simulink library "AtomicLibrary"
PostLoadFcn:
  | PacketBusGenerator; RailCabBusGenerator
(part 1 of 8)

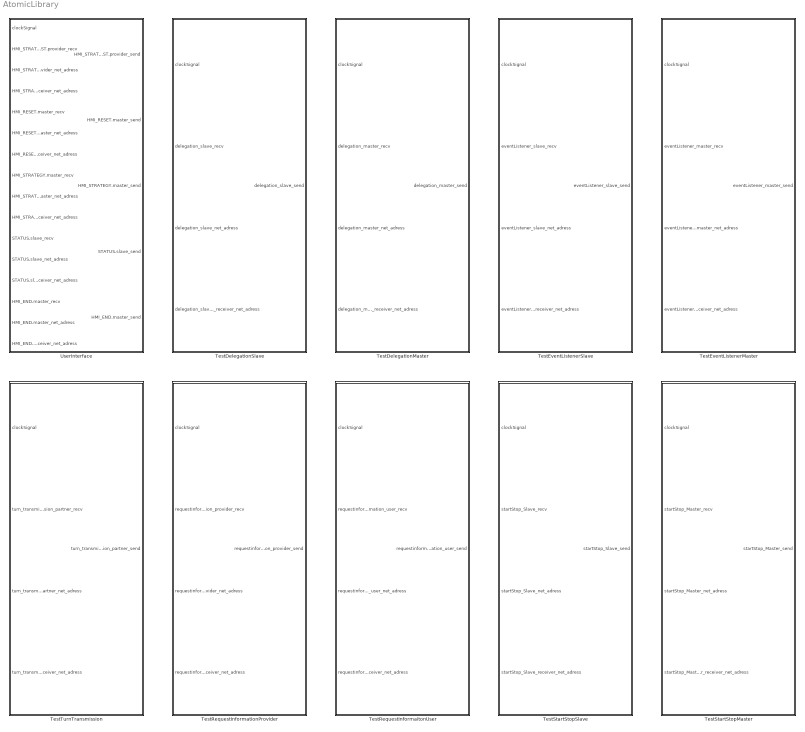
== system AtomicLibrary ==
  UserInterface : Subsystem  Tag=id=_qU3SQPdmEeGH_6eRdlYQdA
  TestDelegationSlave : Subsystem  Tag=id=_qXBOYPdmEeGH_6eRdlYQdA
  TestDelegationMaster : Subsystem  Tag=id=_qXK_YPdmEeGH_6eRdlYQdA
  TestEventListenerSlave : Subsystem  Tag=id=_qXV-gPdmEeGH_6eRdlYQdA
  TestEventListenerMaster : Subsystem  Tag=id=_qXgWkPdmEeGH_6eRdlYQdA
  TestTurnTransmission : Subsystem  Tag=id=_qXqHkPdmEeGH_6eRdlYQdA
  TestRequestInformationProvider : Subsystem  Tag=id=_qX1GsPdmEeGH_6eRdlYQdA
  TestRequestInformaitonUser : Subsystem  Tag=id=_qX_ewPdmEeGH_6eRdlYQdA
  TestStartStopSlave : Subsystem  Tag=id=_qYNhMPdmEeGH_6eRdlYQdA
  TestStartStopMaster : Subsystem  Tag=id=_qYYgUPdmEeGH_6eRdlYQdA

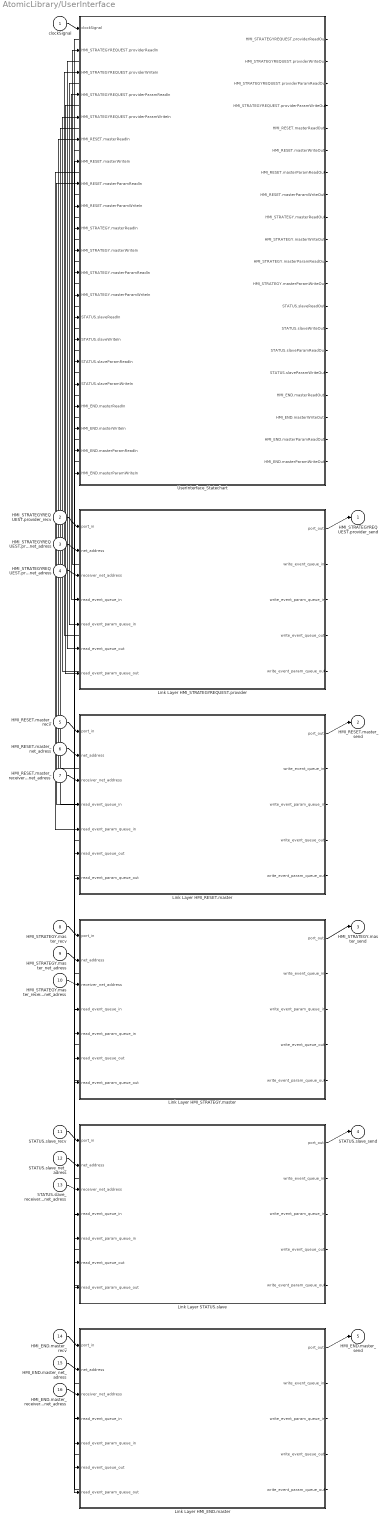
== system AtomicLibrary/UserInterface ==
  clockSignal : Inport  Tag=id=_qWKSwPdmEeGH_6eRdlYQdA  Port=1  DataType=auto  OutDataType=fixdt(1, 16)  OutScaling=2^0  OutDataTypeStr=Inherit: auto
  HMI_STRATEGYREQUEST.provider_recv : Inport  Tag=id=_r0Kh0PdmEeGH_6eRdlYQdA  Port=2  DataType=auto  OutDataType=fixdt(1, 16)  OutScaling=2^0  OutDataTypeStr=Inherit: auto
  HMI_STRATEGYREQUEST.provider_net_adress : Inport  Tag=id=_r0M-EPdmEeGH_6eRdlYQdA  Port=3  DataType=auto  OutDataType=fixdt(1, 16)  OutScaling=2^0  OutDataTypeStr=Inherit: auto
  HMI_STRATEGYREQUEST.provider_receiver_net_adress : Inport  Tag=id=_r0NlIPdmEeGH_6eRdlYQdA  Port=4  DataType=auto  OutDataType=fixdt(1, 16)  OutScaling=2^0  OutDataTypeStr=Inherit: auto
  HMI_RESET.master_recv : Inport  Tag=id=_r-XmsPdmEeGH_6eRdlYQdA  Port=5  DataType=auto  OutDataType=fixdt(1, 16)  OutScaling=2^0  OutDataTypeStr=Inherit: auto
  HMI_RESET.master_net_adress : Inport  Tag=id=_r-aC8PdmEeGH_6eRdlYQdA  Port=6  DataType=auto  OutDataType=fixdt(1, 16)  OutScaling=2^0  OutDataTypeStr=Inherit: auto
  HMI_RESET.master_receiver_net_adress : Inport  Tag=id=_r-aqAPdmEeGH_6eRdlYQdA  Port=7  DataType=auto  OutDataType=fixdt(1, 16)  OutScaling=2^0  OutDataTypeStr=Inherit: auto
  HMI_STRATEGY.master_recv : Inport  Tag=id=_sId94PdmEeGH_6eRdlYQdA  Port=8  DataType=auto  OutDataType=fixdt(1, 16)  OutScaling=2^0  OutDataTypeStr=Inherit: auto
  HMI_STRATEGY.master_net_adress : Inport  Tag=id=_sIhoQPdmEeGH_6eRdlYQdA  Port=9  DataType=auto  OutDataType=fixdt(1, 16)  OutScaling=2^0  OutDataTypeStr=Inherit: auto
  HMI_STRATEGY.master_receiver_net_adress : Inport  Tag=id=_sIi2YPdmEeGH_6eRdlYQdA  Port=10  DataType=auto  OutDataType=fixdt(1, 16)  OutScaling=2^0  OutDataTypeStr=Inherit: auto
  STATUS.slave_recv : Inport  Tag=id=_sS5sQPdmEeGH_6eRdlYQdA  Port=11  DataType=auto  OutDataType=fixdt(1, 16)  OutScaling=2^0  OutDataTypeStr=Inherit: auto
  STATUS.slave_net_adress : Inport  Tag=id=_sS8vkPdmEeGH_6eRdlYQdA  Port=12  DataType=auto  OutDataType=fixdt(1, 16)  OutScaling=2^0  OutDataTypeStr=Inherit: auto
  STATUS.slave_receiver_net_adress : Inport  Tag=id=_sS9WoPdmEeGH_6eRdlYQdA  Port=13  DataType=auto  OutDataType=fixdt(1, 16)  OutScaling=2^0  OutDataTypeStr=Inherit: auto
  HMI_END.master_recv : Inport  Tag=id=_sc4usPdmEeGH_6eRdlYQdA  Port=14  DataType=auto  OutDataType=fixdt(1, 16)  OutScaling=2^0  OutDataTypeStr=Inherit: auto
  HMI_END.master_net_adress : Inport  Tag=id=_sc7K8PdmEeGH_6eRdlYQdA  Port=15  DataType=auto  OutDataType=fixdt(1, 16)  OutScaling=2^0  OutDataTypeStr=Inherit: auto
  HMI_END.master_receiver_net_adress : Inport  Tag=id=_sc7yAPdmEeGH_6eRdlYQdA  Port=16  DataType=auto  OutDataType=fixdt(1, 16)  OutScaling=2^0  OutDataTypeStr=Inherit: auto
  HMI_STRATEGYREQUEST.provider_send : Outport  Tag=id=_r0J6wPdmEeGH_6eRdlYQdA  Port=1  DataType=auto  OutDataType=fixdt(1, 16)  OutScaling=2^0  OutDataTypeStr=Inherit: auto
  HMI_RESET.master_send : Outport  Tag=id=_r-W_oPdmEeGH_6eRdlYQdA  Port=2  DataType=auto  OutDataType=fixdt(1, 16)  OutScaling=2^0  OutDataTypeStr=Inherit: auto
  HMI_STRATEGY.master_send : Outport  Tag=id=_sIcvwPdmEeGH_6eRdlYQdA  Port=3  DataType=auto  OutDataType=fixdt(1, 16)  OutScaling=2^0  OutDataTypeStr=Inherit: auto
  STATUS.slave_send : Outport  Tag=id=_sS5FMPdmEeGH_6eRdlYQdA  Port=4  DataType=auto  OutDataType=fixdt(1, 16)  OutScaling=2^0  OutDataTypeStr=Inherit: auto
  HMI_END.master_send : Outport  Tag=id=_sc4HoPdmEeGH_6eRdlYQdA  Port=5  DataType=auto  OutDataType=fixdt(1, 16)  OutScaling=2^0  OutDataTypeStr=Inherit: auto
  Link Layer HMI_STRATEGYREQUEST.provider : Subsystem  Tag=id=_r0MXBPdmEeGH_6eRdlYQdA
  Link Layer HMI_RESET.master : Subsystem  Tag=id=_r-Zb4_dmEeGH_6eRdlYQdA
  Link Layer HMI_STRATEGY.master : Subsystem  Tag=id=_sIgaIfdmEeGH_6eRdlYQdA
  Link Layer STATUS.slave : Subsystem  Tag=id=_sS7hdPdmEeGH_6eRdlYQdA
  Link Layer HMI_END.master : Subsystem  Tag=id=_sc6j4fdmEeGH_6eRdlYQdA
  UserInterface_Statechart : Stateflow chart  Tag=id=_qVXokPdmEeGH_6eRdlYQdA
  wires:
  clockSignal/1 -> UserInterface_Statechart/1(clockSignal)
  Link Layer HMI_STRATEGYREQUEST.provider/1(port_out) -> HMI_STRATEGYREQUEST.provider_send/1
  HMI_STRATEGYREQUEST.provider_recv/1 -> Link Layer HMI_STRATEGYREQUEST.provider/1(port_in)
  UserInterface_Statechart/1(HMI_STRATEGYREQUEST.providerReadOut) -> Link Layer HMI_STRATEGYREQUEST.provider/4(read_event_queue_in)
  Link Layer HMI_STRATEGYREQUEST.provider/2(write_event_queue_in) -> UserInterface_Statechart/2(HMI_STRATEGYREQUEST.providerReadIn)
  Link Layer HMI_STRATEGYREQUEST.provider/3(write_event_param_queue_in) -> UserInterface_Statechart/4(HMI_STRATEGYREQUEST.providerParamReadIn)
  UserInterface_Statechart/3(HMI_STRATEGYREQUEST.providerParamReadOut) -> Link Layer HMI_STRATEGYREQUEST.provider/5(read_event_param_queue_in)
  UserInterface_Statechart/2(HMI_STRATEGYREQUEST.providerWriteOut) -> Link Layer HMI_STRATEGYREQUEST.provider/6(read_event_queue_out)
  UserInterface_Statechart/4(HMI_STRATEGYREQUEST.providerParamWriteOut) -> Link Layer HMI_STRATEGYREQUEST.provider/7(read_event_param_queue_out)
  Link Layer HMI_STRATEGYREQUEST.provider/4(write_event_queue_out) -> UserInterface_Statechart/3(HMI_STRATEGYREQUEST.providerWriteIn)
  Link Layer HMI_STRATEGYREQUEST.provider/5(write_event_param_queue_out) -> UserInterface_Statechart/5(HMI_STRATEGYREQUEST.providerParamWriteIn)
  HMI_STRATEGYREQUEST.provider_net_adress/1 -> Link Layer HMI_STRATEGYREQUEST.provider/2(net_address)
  HMI_STRATEGYREQUEST.provider_receiver_net_adress/1 -> Link Layer HMI_STRATEGYREQUEST.provider/3(receiver_net_address)
  Link Layer HMI_RESET.master/1(port_out) -> HMI_RESET.master_send/1
  HMI_RESET.master_recv/1 -> Link Layer HMI_RESET.master/1(port_in)
  UserInterface_Statechart/5(HMI_RESET.masterReadOut) -> Link Layer HMI_RESET.master/4(read_event_queue_in)
  Link Layer HMI_RESET.master/2(write_event_queue_in) -> UserInterface_Statechart/6(HMI_RESET.masterReadIn)
  Link Layer HMI_RESET.master/3(write_event_param_queue_in) -> UserInterface_Statechart/8(HMI_RESET.masterParamReadIn)
  UserInterface_Statechart/7(HMI_RESET.masterParamReadOut) -> Link Layer HMI_RESET.master/5(read_event_param_queue_in)
  UserInterface_Statechart/6(HMI_RESET.masterWriteOut) -> Link Layer HMI_RESET.master/6(read_event_queue_out)
  UserInterface_Statechart/8(HMI_RESET.masterParamWriteOut) -> Link Layer HMI_RESET.master/7(read_event_param_queue_out)
  Link Layer HMI_RESET.master/4(write_event_queue_out) -> UserInterface_Statechart/7(HMI_RESET.masterWriteIn)
  Link Layer HMI_RESET.master/5(write_event_param_queue_out) -> UserInterface_Statechart/9(HMI_RESET.masterParamWriteIn)
  HMI_RESET.master_net_adress/1 -> Link Layer HMI_RESET.master/2(net_address)
  HMI_RESET.master_receiver_net_adress/1 -> Link Layer HMI_RESET.master/3(receiver_net_address)
  Link Layer HMI_STRATEGY.master/1(port_out) -> HMI_STRATEGY.master_send/1
  HMI_STRATEGY.master_recv/1 -> Link Layer HMI_STRATEGY.master/1(port_in)
  UserInterface_Statechart/9(HMI_STRATEGY.masterReadOut) -> Link Layer HMI_STRATEGY.master/4(read_event_queue_in)
  Link Layer HMI_STRATEGY.master/2(write_event_queue_in) -> UserInterface_Statechart/10(HMI_STRATEGY.masterReadIn)
  Link Layer HMI_STRATEGY.master/3(write_event_param_queue_in) -> UserInterface_Statechart/12(HMI_STRATEGY.masterParamReadIn)
  UserInterface_Statechart/11(HMI_STRATEGY.masterParamReadOut) -> Link Layer HMI_STRATEGY.master/5(read_event_param_queue_in)
  UserInterface_Statechart/10(HMI_STRATEGY.masterWriteOut) -> Link Layer HMI_STRATEGY.master/6(read_event_queue_out)
  UserInterface_Statechart/12(HMI_STRATEGY.masterParamWriteOut) -> Link Layer HMI_STRATEGY.master/7(read_event_param_queue_out)
  Link Layer HMI_STRATEGY.master/4(write_event_queue_out) -> UserInterface_Statechart/11(HMI_STRATEGY.masterWriteIn)
  Link Layer HMI_STRATEGY.master/5(write_event_param_queue_out) -> UserInterface_Statechart/13(HMI_STRATEGY.masterParamWriteIn)
  HMI_STRATEGY.master_net_adress/1 -> Link Layer HMI_STRATEGY.master/2(net_address)
  HMI_STRATEGY.master_receiver_net_adress/1 -> Link Layer HMI_STRATEGY.master/3(receiver_net_address)
  Link Layer STATUS.slave/1(port_out) -> STATUS.slave_send/1
  STATUS.slave_recv/1 -> Link Layer STATUS.slave/1(port_in)
  UserInterface_Statechart/13(STATUS.slaveReadOut) -> Link Layer STATUS.slave/4(read_event_queue_in)
  Link Layer STATUS.slave/2(write_event_queue_in) -> UserInterface_Statechart/14(STATUS.slaveReadIn)
  Link Layer STATUS.slave/3(write_event_param_queue_in) -> UserInterface_Statechart/16(STATUS.slaveParamReadIn)
  UserInterface_Statechart/15(STATUS.slaveParamReadOut) -> Link Layer STATUS.slave/5(read_event_param_queue_in)
  UserInterface_Statechart/14(STATUS.slaveWriteOut) -> Link Layer STATUS.slave/6(read_event_queue_out)
  UserInterface_Statechart/16(STATUS.slaveParamWriteOut) -> Link Layer STATUS.slave/7(read_event_param_queue_out)
  Link Layer STATUS.slave/4(write_event_queue_out) -> UserInterface_Statechart/15(STATUS.slaveWriteIn)
  Link Layer STATUS.slave/5(write_event_param_queue_out) -> UserInterface_Statechart/17(STATUS.slaveParamWriteIn)
  STATUS.slave_net_adress/1 -> Link Layer STATUS.slave/2(net_address)
  STATUS.slave_receiver_net_adress/1 -> Link Layer STATUS.slave/3(receiver_net_address)
  Link Layer HMI_END.master/1(port_out) -> HMI_END.master_send/1
  HMI_END.master_recv/1 -> Link Layer HMI_END.master/1(port_in)
  UserInterface_Statechart/17(HMI_END.masterReadOut) -> Link Layer HMI_END.master/4(read_event_queue_in)
  Link Layer HMI_END.master/2(write_event_queue_in) -> UserInterface_Statechart/18(HMI_END.masterReadIn)
  Link Layer HMI_END.master/3(write_event_param_queue_in) -> UserInterface_Statechart/20(HMI_END.masterParamReadIn)
  UserInterface_Statechart/19(HMI_END.masterParamReadOut) -> Link Layer HMI_END.master/5(read_event_param_queue_in)
  UserInterface_Statechart/18(HMI_END.masterWriteOut) -> Link Layer HMI_END.master/6(read_event_queue_out)
  UserInterface_Statechart/20(HMI_END.masterParamWriteOut) -> Link Layer HMI_END.master/7(read_event_param_queue_out)
  Link Layer HMI_END.master/4(write_event_queue_out) -> UserInterface_Statechart/19(HMI_END.masterWriteIn)
  Link Layer HMI_END.master/5(write_event_param_queue_out) -> UserInterface_Statechart/21(HMI_END.masterParamWriteIn)
  HMI_END.master_net_adress/1 -> Link Layer HMI_END.master/2(net_address)
  HMI_END.master_receiver_net_adress/1 -> Link Layer HMI_END.master/3(receiver_net_address)

== system AtomicLibrary/TestDelegationSlave ==
  clockSignal : Inport  Tag=id=_qXCcgfdmEeGH_6eRdlYQdA  Port=1  DataType=auto  OutDataType=fixdt(1, 16)  OutScaling=2^0  OutDataTypeStr=Inherit: auto
  delegation_slave_recv : Inport  Tag=id=_qhxF0PdmEeGH_6eRdlYQdA  Port=2  DataType=auto  OutDataType=fixdt(1, 16)  OutScaling=2^0  OutDataTypeStr=Inherit: auto
  delegation_slave_net_adress : Inport  Tag=id=_qhziEPdmEeGH_6eRdlYQdA  Port=3  DataType=auto  OutDataType=fixdt(1, 16)  OutScaling=2^0  OutDataTypeStr=Inherit: auto
  delegation_slave_receiver_net_adress : Inport  Tag=id=_qh0JIPdmEeGH_6eRdlYQdA  Port=4  DataType=auto  OutDataType=fixdt(1, 16)  OutScaling=2^0  OutDataTypeStr=Inherit: auto
  delegation_slave_send : Outport  Tag=id=_qhwewPdmEeGH_6eRdlYQdA  Port=1  DataType=auto  OutDataType=fixdt(1, 16)  OutScaling=2^0  OutDataTypeStr=Inherit: auto
  Link Layer delegation_slave : Subsystem  Tag=id=_qhy7A_dmEeGH_6eRdlYQdA
  TestDelegationSlave_Statechart : Stateflow chart  Tag=id=_qXB1cPdmEeGH_6eRdlYQdA
  wires:
  clockSignal/1 -> TestDelegationSlave_Statechart/1(clockSignal)
  Link Layer delegation_slave/1(port_out) -> delegation_slave_send/1
  delegation_slave_recv/1 -> Link Layer delegation_slave/1(port_in)
  TestDelegationSlave_Statechart/1(delegation_slaveReadOut) -> Link Layer delegation_slave/4(read_event_queue_in)
  Link Layer delegation_slave/2(write_event_queue_in) -> TestDelegationSlave_Statechart/2(delegation_slaveReadIn)
  Link Layer delegation_slave/3(write_event_param_queue_in) -> TestDelegationSlave_Statechart/4(delegation_slaveParamReadIn)
  TestDelegationSlave_Statechart/3(delegation_slaveParamReadOut) -> Link Layer delegation_slave/5(read_event_param_queue_in)
  TestDelegationSlave_Statechart/2(delegation_slaveWriteOut) -> Link Layer delegation_slave/6(read_event_queue_out)
  TestDelegationSlave_Statechart/4(delegation_slaveParamWriteOut) -> Link Layer delegation_slave/7(read_event_param_queue_out)
  Link Layer delegation_slave/4(write_event_queue_out) -> TestDelegationSlave_Statechart/3(delegation_slaveWriteIn)
  Link Layer delegation_slave/5(write_event_param_queue_out) -> TestDelegationSlave_Statechart/5(delegation_slaveParamWriteIn)
  delegation_slave_net_adress/1 -> Link Layer delegation_slave/2(net_address)
  delegation_slave_receiver_net_adress/1 -> Link Layer delegation_slave/3(receiver_net_address)

== system AtomicLibrary/TestDelegationMaster ==
  clockSignal : Inport  Tag=id=_qXMNgfdmEeGH_6eRdlYQdA  Port=1  DataType=auto  OutDataType=fixdt(1, 16)  OutScaling=2^0  OutDataTypeStr=Inherit: auto
  delegation_master_recv : Inport  Tag=id=_qrRnIPdmEeGH_6eRdlYQdA  Port=2  DataType=auto  OutDataType=fixdt(1, 16)  OutScaling=2^0  OutDataTypeStr=Inherit: auto
  delegation_master_net_adress : Inport  Tag=id=_qrUDYPdmEeGH_6eRdlYQdA  Port=3  DataType=auto  OutDataType=fixdt(1, 16)  OutScaling=2^0  OutDataTypeStr=Inherit: auto
  delegation_master_receiver_net_adress : Inport  Tag=id=_qrUqcPdmEeGH_6eRdlYQdA  Port=4  DataType=auto  OutDataType=fixdt(1, 16)  OutScaling=2^0  OutDataTypeStr=Inherit: auto
  delegation_master_send : Outport  Tag=id=_qrRAEPdmEeGH_6eRdlYQdA  Port=1  DataType=auto  OutDataType=fixdt(1, 16)  OutScaling=2^0  OutDataTypeStr=Inherit: auto
  Link Layer delegation_master : Subsystem  Tag=id=_qrTcU_dmEeGH_6eRdlYQdA
  TestDelegationMaster_Statechart : Stateflow chart  Tag=id=_qXLmcPdmEeGH_6eRdlYQdA
  wires:
  clockSignal/1 -> TestDelegationMaster_Statechart/1(clockSignal)
  Link Layer delegation_master/1(port_out) -> delegation_master_send/1
  delegation_master_recv/1 -> Link Layer delegation_master/1(port_in)
  TestDelegationMaster_Statechart/1(delegation_masterReadOut) -> Link Layer delegation_master/4(read_event_queue_in)
  Link Layer delegation_master/2(write_event_queue_in) -> TestDelegationMaster_Statechart/2(delegation_masterReadIn)
  Link Layer delegation_master/3(write_event_param_queue_in) -> TestDelegationMaster_Statechart/4(delegation_masterParamReadIn)
  TestDelegationMaster_Statechart/3(delegation_masterParamReadOut) -> Link Layer delegation_master/5(read_event_param_queue_in)
  TestDelegationMaster_Statechart/2(delegation_masterWriteOut) -> Link Layer delegation_master/6(read_event_queue_out)
  TestDelegationMaster_Statechart/4(delegation_masterParamWriteOut) -> Link Layer delegation_master/7(read_event_param_queue_out)
  Link Layer delegation_master/4(write_event_queue_out) -> TestDelegationMaster_Statechart/3(delegation_masterWriteIn)
  Link Layer delegation_master/5(write_event_param_queue_out) -> TestDelegationMaster_Statechart/5(delegation_masterParamWriteIn)
  delegation_master_net_adress/1 -> Link Layer delegation_master/2(net_address)
  delegation_master_receiver_net_adress/1 -> Link Layer delegation_master/3(receiver_net_address)

== system AtomicLibrary/TestEventListenerSlave ==
  clockSignal : Inport  Tag=id=_qXXMofdmEeGH_6eRdlYQdA  Port=1  DataType=auto  OutDataType=fixdt(1, 16)  OutScaling=2^0  OutDataTypeStr=Inherit: auto
  eventListener_slave_recv : Inport  Tag=id=_q0bjIPdmEeGH_6eRdlYQdA  Port=2  DataType=auto  OutDataType=fixdt(1, 16)  OutScaling=2^0  OutDataTypeStr=Inherit: auto
  eventListener_slave_net_adress : Inport  Tag=id=_q0d_YPdmEeGH_6eRdlYQdA  Port=3  DataType=auto  OutDataType=fixdt(1, 16)  OutScaling=2^0  OutDataTypeStr=Inherit: auto
  eventListener_slave_receiver_net_adress : Inport  Tag=id=_q0d_YfdmEeGH_6eRdlYQdA  Port=4  DataType=auto  OutDataType=fixdt(1, 16)  OutScaling=2^0  OutDataTypeStr=Inherit: auto
  eventListener_slave_send : Outport  Tag=id=_q0a8EPdmEeGH_6eRdlYQdA  Port=1  DataType=auto  OutDataType=fixdt(1, 16)  OutScaling=2^0  OutDataTypeStr=Inherit: auto
  Link Layer eventListener_slave : Subsystem  Tag=id=_q0dYUPdmEeGH_6eRdlYQdA
  TestEventListenerSlave_Statechart : Stateflow chart  Tag=id=_qXWlkPdmEeGH_6eRdlYQdA
  wires:
  clockSignal/1 -> TestEventListenerSlave_Statechart/1(clockSignal)
  Link Layer eventListener_slave/1(port_out) -> eventListener_slave_send/1
  eventListener_slave_recv/1 -> Link Layer eventListener_slave/1(port_in)
  TestEventListenerSlave_Statechart/1(eventListener_slaveReadOut) -> Link Layer eventListener_slave/4(read_event_queue_in)
  Link Layer eventListener_slave/2(write_event_queue_in) -> TestEventListenerSlave_Statechart/2(eventListener_slaveReadIn)
  Link Layer eventListener_slave/3(write_event_param_queue_in) -> TestEventListenerSlave_Statechart/4(eventListener_slaveParamReadIn)
  TestEventListenerSlave_Statechart/3(eventListener_slaveParamReadOut) -> Link Layer eventListener_slave/5(read_event_param_queue_in)
  TestEventListenerSlave_Statechart/2(eventListener_slaveWriteOut) -> Link Layer eventListener_slave/6(read_event_queue_out)
  TestEventListenerSlave_Statechart/4(eventListener_slaveParamWriteOut) -> Link Layer eventListener_slave/7(read_event_param_queue_out)
  Link Layer eventListener_slave/4(write_event_queue_out) -> TestEventListenerSlave_Statechart/3(eventListener_slaveWriteIn)
  Link Layer eventListener_slave/5(write_event_param_queue_out) -> TestEventListenerSlave_Statechart/5(eventListener_slaveParamWriteIn)
  eventListener_slave_net_adress/1 -> Link Layer eventListener_slave/2(net_address)
  eventListener_slave_receiver_net_adress/1 -> Link Layer eventListener_slave/3(receiver_net_address)

== system AtomicLibrary/TestEventListenerMaster ==
  clockSignal : Inport  Tag=id=_qXg9ovdmEeGH_6eRdlYQdA  Port=1  DataType=auto  OutDataType=fixdt(1, 16)  OutScaling=2^0  OutDataTypeStr=Inherit: auto
  eventListener_master_recv : Inport  Tag=id=_q9nUUPdmEeGH_6eRdlYQdA  Port=2  DataType=auto  OutDataType=fixdt(1, 16)  OutScaling=2^0  OutDataTypeStr=Inherit: auto
  eventListener_master_net_adress : Inport  Tag=id=_q9pJgPdmEeGH_6eRdlYQdA  Port=3  DataType=auto  OutDataType=fixdt(1, 16)  OutScaling=2^0  OutDataTypeStr=Inherit: auto
  eventListener_master_receiver_net_adress : Inport  Tag=id=_q9pwkPdmEeGH_6eRdlYQdA  Port=4  DataType=auto  OutDataType=fixdt(1, 16)  OutScaling=2^0  OutDataTypeStr=Inherit: auto
  eventListener_master_send : Outport  Tag=id=_q9mtQPdmEeGH_6eRdlYQdA  Port=1  DataType=auto  OutDataType=fixdt(1, 16)  OutScaling=2^0  OutDataTypeStr=Inherit: auto
  Link Layer eventListener_master : Subsystem  Tag=id=_q9oidfdmEeGH_6eRdlYQdA
  TestEventListenerMaster_Statechart : Stateflow chart  Tag=id=_qXg9oPdmEeGH_6eRdlYQdA
  wires:
  clockSignal/1 -> TestEventListenerMaster_Statechart/1(clockSignal)
  Link Layer eventListener_master/1(port_out) -> eventListener_master_send/1
  eventListener_master_recv/1 -> Link Layer eventListener_master/1(port_in)
  TestEventListenerMaster_Statechart/1(eventListener_masterReadOut) -> Link Layer eventListener_master/4(read_event_queue_in)
  Link Layer eventListener_master/2(write_event_queue_in) -> TestEventListenerMaster_Statechart/2(eventListener_masterReadIn)
  Link Layer eventListener_master/3(write_event_param_queue_in) -> TestEventListenerMaster_Statechart/4(eventListener_masterParamReadIn)
  TestEventListenerMaster_Statechart/3(eventListener_masterParamReadOut) -> Link Layer eventListener_master/5(read_event_param_queue_in)
  TestEventListenerMaster_Statechart/2(eventListener_masterWriteOut) -> Link Layer eventListener_master/6(read_event_queue_out)
  TestEventListenerMaster_Statechart/4(eventListener_masterParamWriteOut) -> Link Layer eventListener_master/7(read_event_param_queue_out)
  Link Layer eventListener_master/4(write_event_queue_out) -> TestEventListenerMaster_Statechart/3(eventListener_masterWriteIn)
  Link Layer eventListener_master/5(write_event_param_queue_out) -> TestEventListenerMaster_Statechart/5(eventListener_masterParamWriteIn)
  eventListener_master_net_adress/1 -> Link Layer eventListener_master/2(net_address)
  eventListener_master_receiver_net_adress/1 -> Link Layer eventListener_master/3(receiver_net_address)

== system AtomicLibrary/TestTurnTransmission ==
  clockSignal : Inport  Tag=id=_qXrVsfdmEeGH_6eRdlYQdA  Port=1  DataType=auto  OutDataType=fixdt(1, 16)  OutScaling=2^0  OutDataTypeStr=Inherit: auto
  turn_transmission_partner_recv : Inport  Tag=id=_rGbSEPdmEeGH_6eRdlYQdA  Port=2  DataType=auto  OutDataType=fixdt(1, 16)  OutScaling=2^0  OutDataTypeStr=Inherit: auto
  turn_transmission_partner_net_adress : Inport  Tag=id=_rGduUPdmEeGH_6eRdlYQdA  Port=3  DataType=auto  OutDataType=fixdt(1, 16)  OutScaling=2^0  OutDataTypeStr=Inherit: auto
  turn_transmission_partner_receiver_net_adress : Inport  Tag=id=_rGeVYPdmEeGH_6eRdlYQdA  Port=4  DataType=auto  OutDataType=fixdt(1, 16)  OutScaling=2^0  OutDataTypeStr=Inherit: auto
  turn_transmission_partner_send : Outport  Tag=id=_rGarAPdmEeGH_6eRdlYQdA  Port=1  DataType=auto  OutDataType=fixdt(1, 16)  OutScaling=2^0  OutDataTypeStr=Inherit: auto
  Link Layer turn_transmission_partner : Subsystem  Tag=id=_rGdHQvdmEeGH_6eRdlYQdA
  TestTurnTransmission_Statechart : Stateflow chart  Tag=id=_qXquoPdmEeGH_6eRdlYQdA
  wires:
  clockSignal/1 -> TestTurnTransmission_Statechart/1(clockSignal)
  Link Layer turn_transmission_partner/1(port_out) -> turn_transmission_partner_send/1
  turn_transmission_partner_recv/1 -> Link Layer turn_transmission_partner/1(port_in)
  TestTurnTransmission_Statechart/1(turn_transmission_partnerReadOut) -> Link Layer turn_transmission_partner/4(read_event_queue_in)
  Link Layer turn_transmission_partner/2(write_event_queue_in) -> TestTurnTransmission_Statechart/2(turn_transmission_partnerReadIn)
  Link Layer turn_transmission_partner/3(write_event_param_queue_in) -> TestTurnTransmission_Statechart/4(turn_transmission_partnerParamReadIn)
  TestTurnTransmission_Statechart/3(turn_transmission_partnerParamReadOut) -> Link Layer turn_transmission_partner/5(read_event_param_queue_in)
  TestTurnTransmission_Statechart/2(turn_transmission_partnerWriteOut) -> Link Layer turn_transmission_partner/6(read_event_queue_out)
  TestTurnTransmission_Statechart/4(turn_transmission_partnerParamWriteOut) -> Link Layer turn_transmission_partner/7(read_event_param_queue_out)
  Link Layer turn_transmission_partner/4(write_event_queue_out) -> TestTurnTransmission_Statechart/3(turn_transmission_partnerWriteIn)
  Link Layer turn_transmission_partner/5(write_event_param_queue_out) -> TestTurnTransmission_Statechart/5(turn_transmission_partnerParamWriteIn)
  turn_transmission_partner_net_adress/1 -> Link Layer turn_transmission_partner/2(net_address)
  turn_transmission_partner_receiver_net_adress/1 -> Link Layer turn_transmission_partner/3(receiver_net_address)

== system AtomicLibrary/TestRequestInformationProvider ==
  clockSignal : Inport  Tag=id=_qX2U0fdmEeGH_6eRdlYQdA  Port=1  DataType=auto  OutDataType=fixdt(1, 16)  OutScaling=2^0  OutDataTypeStr=Inherit: auto
  requestinformation_provider_recv : Inport  Tag=id=_rPfHcPdmEeGH_6eRdlYQdA  Port=2  DataType=auto  OutDataType=fixdt(1, 16)  OutScaling=2^0  OutDataTypeStr=Inherit: auto
  requestinformation_provider_net_adress : Inport  Tag=id=_rPiKwPdmEeGH_6eRdlYQdA  Port=3  DataType=auto  OutDataType=fixdt(1, 16)  OutScaling=2^0  OutDataTypeStr=Inherit: auto
  requestinformation_provider_receiver_net_adress : Inport  Tag=id=_rPjY4PdmEeGH_6eRdlYQdA  Port=4  DataType=auto  OutDataType=fixdt(1, 16)  OutScaling=2^0  OutDataTypeStr=Inherit: auto
  requestinformation_provider_send : Outport  Tag=id=_rPegYPdmEeGH_6eRdlYQdA  Port=1  DataType=auto  OutDataType=fixdt(1, 16)  OutScaling=2^0  OutDataTypeStr=Inherit: auto
  Link Layer requestinformation_provider : Subsystem  Tag=id=_rPhjsPdmEeGH_6eRdlYQdA
  TestRequestInformationProvider_Statechart : Stateflow chart  Tag=id=_qX1twPdmEeGH_6eRdlYQdA
  wires:
  clockSignal/1 -> TestRequestInformationProvider_Statechart/1(clockSignal)
  Link Layer requestinformation_provider/1(port_out) -> requestinformation_provider_send/1
  requestinformation_provider_recv/1 -> Link Layer requestinformation_provider/1(port_in)
  TestRequestInformationProvider_Statechart/1(requestinformation_providerReadOut) -> Link Layer requestinformation_provider/4(read_event_queue_in)
  Link Layer requestinformation_provider/2(write_event_queue_in) -> TestRequestInformationProvider_Statechart/2(requestinformation_providerReadIn)
  Link Layer requestinformation_provider/3(write_event_param_queue_in) -> TestRequestInformationProvider_Statechart/4(requestinformation_providerParamReadIn)
  TestRequestInformationProvider_Statechart/3(requestinformation_providerParamReadOut) -> Link Layer requestinformation_provider/5(read_event_param_queue_in)
  TestRequestInformationProvider_Statechart/2(requestinformation_providerWriteOut) -> Link Layer requestinformation_provider/6(read_event_queue_out)
  TestRequestInformationProvider_Statechart/4(requestinformation_providerParamWriteOut) -> Link Layer requestinformation_provider/7(read_event_param_queue_out)
  Link Layer requestinformation_provider/4(write_event_queue_out) -> TestRequestInformationProvider_Statechart/3(requestinformation_providerWriteIn)
  Link Layer requestinformation_provider/5(write_event_param_queue_out) -> TestRequestInformationProvider_Statechart/5(requestinformation_providerParamWriteIn)
  requestinformation_provider_net_adress/1 -> Link Layer requestinformation_provider/2(net_address)
  requestinformation_provider_receiver_net_adress/1 -> Link Layer requestinformation_provider/3(receiver_net_address)

== system AtomicLibrary/TestRequestInformaitonUser ==
  clockSignal : Inport  Tag=id=_qYAs4PdmEeGH_6eRdlYQdA  Port=1  DataType=auto  OutDataType=fixdt(1, 16)  OutScaling=2^0  OutDataTypeStr=Inherit: auto
  requestinformation_user_recv : Inport  Tag=id=_rYAxUPdmEeGH_6eRdlYQdA  Port=2  DataType=auto  OutDataType=fixdt(1, 16)  OutScaling=2^0  OutDataTypeStr=Inherit: auto
  requestinformation_user_net_adress : Inport  Tag=id=_rYCmgPdmEeGH_6eRdlYQdA  Port=3  DataType=auto  OutDataType=fixdt(1, 16)  OutScaling=2^0  OutDataTypeStr=Inherit: auto
  requestinformation_user_receiver_net_adress : Inport  Tag=id=_rYDNkPdmEeGH_6eRdlYQdA  Port=4  DataType=auto  OutDataType=fixdt(1, 16)  OutScaling=2^0  OutDataTypeStr=Inherit: auto
  requestinformation_user_send : Outport  Tag=id=_rYAKQPdmEeGH_6eRdlYQdA  Port=1  DataType=auto  OutDataType=fixdt(1, 16)  OutScaling=2^0  OutDataTypeStr=Inherit: auto
  Link Layer requestinformation_user : Subsystem  Tag=id=_rYB_dPdmEeGH_6eRdlYQdA
  TestRequestInformaitonUser_Statechart : Stateflow chart  Tag=id=_qYAF0PdmEeGH_6eRdlYQdA
  wires:
  clockSignal/1 -> TestRequestInformaitonUser_Statechart/1(clockSignal)
  Link Layer requestinformation_user/1(port_out) -> requestinformation_user_send/1
  requestinformation_user_recv/1 -> Link Layer requestinformation_user/1(port_in)
  TestRequestInformaitonUser_Statechart/1(requestinformation_userReadOut) -> Link Layer requestinformation_user/4(read_event_queue_in)
  Link Layer requestinformation_user/2(write_event_queue_in) -> TestRequestInformaitonUser_Statechart/2(requestinformation_userReadIn)
  Link Layer requestinformation_user/3(write_event_param_queue_in) -> TestRequestInformaitonUser_Statechart/4(requestinformation_userParamReadIn)
  TestRequestInformaitonUser_Statechart/3(requestinformation_userParamReadOut) -> Link Layer requestinformation_user/5(read_event_param_queue_in)
  TestRequestInformaitonUser_Statechart/2(requestinformation_userWriteOut) -> Link Layer requestinformation_user/6(read_event_queue_out)
  TestRequestInformaitonUser_Statechart/4(requestinformation_userParamWriteOut) -> Link Layer requestinformation_user/7(read_event_param_queue_out)
  Link Layer requestinformation_user/4(write_event_queue_out) -> TestRequestInformaitonUser_Statechart/3(requestinformation_userWriteIn)
  Link Layer requestinformation_user/5(write_event_param_queue_out) -> TestRequestInformaitonUser_Statechart/5(requestinformation_userParamWriteIn)
  requestinformation_user_net_adress/1 -> Link Layer requestinformation_user/2(net_address)
  requestinformation_user_receiver_net_adress/1 -> Link Layer requestinformation_user/3(receiver_net_address)

== system AtomicLibrary/TestStartStopSlave ==
  clockSignal : Inport  Tag=id=_qYOvUfdmEeGH_6eRdlYQdA  Port=1  DataType=auto  OutDataType=fixdt(1, 16)  OutScaling=2^0  OutDataTypeStr=Inherit: auto
  startStop_Slave_recv : Inport  Tag=id=_rgzg8PdmEeGH_6eRdlYQdA  Port=2  DataType=auto  OutDataType=fixdt(1, 16)  OutScaling=2^0  OutDataTypeStr=Inherit: auto
  startStop_Slave_net_adress : Inport  Tag=id=_rg19MPdmEeGH_6eRdlYQdA  Port=3  DataType=auto  OutDataType=fixdt(1, 16)  OutScaling=2^0  OutDataTypeStr=Inherit: auto
  startStop_Slave_receiver_net_adress : Inport  Tag=id=_rg2kQPdmEeGH_6eRdlYQdA  Port=4  DataType=auto  OutDataType=fixdt(1, 16)  OutScaling=2^0  OutDataTypeStr=Inherit: auto
  startStop_Slave_send : Outport  Tag=id=_rgy54PdmEeGH_6eRdlYQdA  Port=1  DataType=auto  OutDataType=fixdt(1, 16)  OutScaling=2^0  OutDataTypeStr=Inherit: auto
  Link Layer startStop_Slave : Subsystem  Tag=id=_rg1WIvdmEeGH_6eRdlYQdA
  TestStartStopSlave_Statechart : Stateflow chart  Tag=id=_qYOIQPdmEeGH_6eRdlYQdA
  wires:
  clockSignal/1 -> TestStartStopSlave_Statechart/1(clockSignal)
  Link Layer startStop_Slave/1(port_out) -> startStop_Slave_send/1
  startStop_Slave_recv/1 -> Link Layer startStop_Slave/1(port_in)
  TestStartStopSlave_Statechart/1(startStop_SlaveReadOut) -> Link Layer startStop_Slave/4(read_event_queue_in)
  Link Layer startStop_Slave/2(write_event_queue_in) -> TestStartStopSlave_Statechart/2(startStop_SlaveReadIn)
  Link Layer startStop_Slave/3(write_event_param_queue_in) -> TestStartStopSlave_Statechart/4(startStop_SlaveParamReadIn)
  TestStartStopSlave_Statechart/3(startStop_SlaveParamReadOut) -> Link Layer startStop_Slave/5(read_event_param_queue_in)
  TestStartStopSlave_Statechart/2(startStop_SlaveWriteOut) -> Link Layer startStop_Slave/6(read_event_queue_out)
  TestStartStopSlave_Statechart/4(startStop_SlaveParamWriteOut) -> Link Layer startStop_Slave/7(read_event_param_queue_out)
  Link Layer startStop_Slave/4(write_event_queue_out) -> TestStartStopSlave_Statechart/3(startStop_SlaveWriteIn)
  Link Layer startStop_Slave/5(write_event_param_queue_out) -> TestStartStopSlave_Statechart/5(startStop_SlaveParamWriteIn)
  startStop_Slave_net_adress/1 -> Link Layer startStop_Slave/2(net_address)
  startStop_Slave_receiver_net_adress/1 -> Link Layer startStop_Slave/3(receiver_net_address)

== system AtomicLibrary/TestStartStopMaster ==
  clockSignal : Inport  Tag=id=_qYaVgPdmEeGH_6eRdlYQdA  Port=1  DataType=auto  OutDataType=fixdt(1, 16)  OutScaling=2^0  OutDataTypeStr=Inherit: auto
  startStop_Master_recv : Inport  Tag=id=_rqOisPdmEeGH_6eRdlYQdA  Port=2  DataType=auto  OutDataType=fixdt(1, 16)  OutScaling=2^0  OutDataTypeStr=Inherit: auto
  startStop_Master_net_adress : Inport  Tag=id=_rqQ-8PdmEeGH_6eRdlYQdA  Port=3  DataType=auto  OutDataType=fixdt(1, 16)  OutScaling=2^0  OutDataTypeStr=Inherit: auto
  startStop_Master_receiver_net_adress : Inport  Tag=id=_rqRmAPdmEeGH_6eRdlYQdA  Port=4  DataType=auto  OutDataType=fixdt(1, 16)  OutScaling=2^0  OutDataTypeStr=Inherit: auto
  startStop_Master_send : Outport  Tag=id=_rqN7oPdmEeGH_6eRdlYQdA  Port=1  DataType=auto  OutDataType=fixdt(1, 16)  OutScaling=2^0  OutDataTypeStr=Inherit: auto
  Link Layer startStop_Master : Subsystem  Tag=id=_rqQX4_dmEeGH_6eRdlYQdA
  TestStartStopMaster_Statechart : Stateflow chart  Tag=id=_qYZucPdmEeGH_6eRdlYQdA
  wires:
  clockSignal/1 -> TestStartStopMaster_Statechart/1(clockSignal)
  Link Layer startStop_Master/1(port_out) -> startStop_Master_send/1
  startStop_Master_recv/1 -> Link Layer startStop_Master/1(port_in)
  TestStartStopMaster_Statechart/1(startStop_MasterReadOut) -> Link Layer startStop_Master/4(read_event_queue_in)
  Link Layer startStop_Master/2(write_event_queue_in) -> TestStartStopMaster_Statechart/2(startStop_MasterReadIn)
  Link Layer startStop_Master/3(write_event_param_queue_in) -> TestStartStopMaster_Statechart/4(startStop_MasterParamReadIn)
  TestStartStopMaster_Statechart/3(startStop_MasterParamReadOut) -> Link Layer startStop_Master/5(read_event_param_queue_in)
  TestStartStopMaster_Statechart/2(startStop_MasterWriteOut) -> Link Layer startStop_Master/6(read_event_queue_out)
  TestStartStopMaster_Statechart/4(startStop_MasterParamWriteOut) -> Link Layer startStop_Master/7(read_event_param_queue_out)
  Link Layer startStop_Master/4(write_event_queue_out) -> TestStartStopMaster_Statechart/3(startStop_MasterWriteIn)
  Link Layer startStop_Master/5(write_event_param_queue_out) -> TestStartStopMaster_Statechart/5(startStop_MasterParamWriteIn)
  startStop_Master_net_adress/1 -> Link Layer startStop_Master/2(net_address)
  startStop_Master_receiver_net_adress/1 -> Link Layer startStop_Master/3(receiver_net_address)

== system AtomicLibrary/UserInterface/Link Layer HMI_STRATEGYREQUEST.provider ==
  port_in : Inport  Tag=id=_r0aZcPdmEeGH_6eRdlYQdA  Port=1  PortDimensions=-1  DataType=auto  OutDataType=fixdt(1, 16)  OutScaling=2^0  UseBusObject=on  OutDataTypeStr=Inherit: auto
      settings: BusObject=PacketBus
  net_address : Inport  Tag=id=_r0i8UPdmEeGH_6eRdlYQdA  Port=2  PortDimensions=-1  DataType=uint8  OutDataType=fixdt(1, 16)  OutScaling=2^0  OutDataTypeStr=uint8
  receiver_net_address : Inport  Tag=id=_r0kKcPdmEeGH_6eRdlYQdA  Port=3  PortDimensions=-1  DataType=uint8  OutDataType=fixdt(1, 16)  OutScaling=2^0  OutDataTypeStr=uint8
  read_event_queue_in : Inport  Tag=id=_r0bAgPdmEeGH_6eRdlYQdA  Port=4  PortDimensions=-1  DataType=auto  OutDataType=fixdt(1, 16)  OutScaling=2^0  OutDataTypeStr=Inherit: auto
  read_event_param_queue_in : Inport  Tag=id=_r0dcwPdmEeGH_6eRdlYQdA  Port=5  PortDimensions=-1  DataType=auto  OutDataType=fixdt(1, 16)  OutScaling=2^0  OutDataTypeStr=Inherit: auto
  read_event_queue_out : Inport  Tag=id=_r0eD0PdmEeGH_6eRdlYQdA  Port=6  PortDimensions=-1  DataType=auto  OutDataType=fixdt(1, 16)  OutScaling=2^0  OutDataTypeStr=Inherit: auto
  read_event_param_queue_out : Inport  Tag=id=_r0fR8PdmEeGH_6eRdlYQdA  Port=7  PortDimensions=-1  DataType=auto  OutDataType=fixdt(1, 16)  OutScaling=2^0  OutDataTypeStr=Inherit: auto
  port_out : Outport  Tag=id=_r0ZyYfdmEeGH_6eRdlYQdA  Port=1  PortDimensions=-1  DataType=auto  OutDataType=fixdt(1, 16)  OutScaling=2^0  UseBusObject=on  OutDataTypeStr=Inherit: auto
      settings: BusObject=PacketBus
  write_event_queue_in : Outport  Tag=id=_r0cOoPdmEeGH_6eRdlYQdA  Port=2  PortDimensions=-1  DataType=auto  OutDataType=fixdt(1, 16)  OutScaling=2^0  OutDataTypeStr=Inherit: auto
  write_event_param_queue_in : Outport  Tag=id=_r0c1sPdmEeGH_6eRdlYQdA  Port=3  PortDimensions=-1  DataType=auto  OutDataType=fixdt(1, 16)  OutScaling=2^0  OutDataTypeStr=Inherit: auto
  write_event_queue_out : Outport  Tag=id=_r0ggEPdmEeGH_6eRdlYQdA  Port=4  PortDimensions=-1  DataType=auto  OutDataType=fixdt(1, 16)  OutScaling=2^0  OutDataTypeStr=Inherit: auto
  write_event_param_queue_out : Outport  Tag=id=_r0huMPdmEeGH_6eRdlYQdA  Port=5  PortDimensions=-1  DataType=auto  OutDataType=fixdt(1, 16)  OutScaling=2^0  OutDataTypeStr=Inherit: auto
  DataLinkLayer : Subsystem  Tag=id=_r0l_ofdmEeGH_6eRdlYQdA
  Bus Selector : BusSelector  OutputSignals=from,to,msg,param,pkgid,time  Tag=id=_r0lYkPdmEeGH_6eRdlYQdA
  Unit Delay1 : UnitDelay  Tag=id=_r0lYkfdmEeGH_6eRdlYQdA  SampleTime=-1
  Unit Delay2 : UnitDelay  Tag=id=_r0l_oPdmEeGH_6eRdlYQdA  SampleTime=-1
  Unit Delay3 : UnitDelay  Tag=id=_r0mmsPdmEeGH_6eRdlYQdA  SampleTime=-1
  Bus Creator : BusCreator  Inputs=6  UseBusObject=on  Tag=id=_r0nNwPdmEeGH_6eRdlYQdA
      settings: BusObject=PacketBus
  Unit Delay4 : UnitDelay  Tag=id=_r0n00PdmEeGH_6eRdlYQdA  SampleTime=-1
  Terminator : Terminator
      settings: Tag=id=_r0n00fdmEeGH_6eRdlYQdA
  Receive Packet : Stateflow chart  Tag=id=_r0n00vdmEeGH_6eRdlYQdA
  Send Packet : Stateflow chart  Tag=id=_r0ob4PdmEeGH_6eRdlYQdA
  wires:
  DataLinkLayer/3(snd_msg_out) -> Bus Creator/3
  DataLinkLayer/8(recv_msg_out) -> Receive Packet/2(packetMsg)
  Send Packet/3(eventQueue) -> Unit Delay1/1
  DataLinkLayer/7(recv_from_out) -> Receive Packet/1(packetFrom)
  Bus Selector/3 -> DataLinkLayer/3(recv_msg_in)
  read_event_param_queue_in/1 -> Receive Packet/5(eventParamQueueIn)
  Receive Packet/3(bufferOverflow) -> Terminator/1
  receiver_net_address/1 -> DataLinkLayer/8(snd_to_in)
  Receive Packet/2(eventParamQueue) -> Unit Delay4/1
  read_event_queue_out/1 -> Send Packet/2(eventQueueIn)
  DataLinkLayer/9(recv_param_out) -> Receive Packet/3(packetParam)
  Send Packet/2(packetParam) -> DataLinkLayer/10(snd_param_in)
  Bus Selector/2 -> DataLinkLayer/2(recv_to_in)
  port_in/1 -> Bus Selector/1
  read_event_param_queue_out/1 -> Send Packet/3(eventParamQueueIn)
  Send Packet/4(eventParamQueue) -> Unit Delay2/1
  Bus Selector/5 -> DataLinkLayer/5(recv_pkgid_in)
  Unit Delay4/1 -> write_event_param_queue_in/1
  read_event_queue_in/1 -> Receive Packet/4(eventQueueIn)
  Bus Selector/4 -> DataLinkLayer/4(recv_param_in)
  DataLinkLayer/2(snd_to_out) -> Bus Creator/2
  Bus Selector/6 -> DataLinkLayer/6(recv_time_in), Send Packet/1(busSizeSignal)
  Receive Packet/1(eventQueue) -> Unit Delay3/1
  DataLinkLayer/6(snd_time_out) -> Bus Creator/6
  Unit Delay1/1 -> write_event_queue_out/1
  DataLinkLayer/1(snd_from_out) -> Bus Creator/1
  DataLinkLayer/5(snd_pkgid_out) -> Bus Creator/5
  net_address/1 -> DataLinkLayer/7(snd_from_in)
  Send Packet/1(packetMsg) -> DataLinkLayer/9(snd_msg_in)
  Bus Creator/1 -> port_out/1  "Outport11"
  Unit Delay3/1 -> write_event_queue_in/1
  Bus Selector/1 -> DataLinkLayer/1(recv_from_in)
  Unit Delay2/1 -> write_event_param_queue_out/1
  DataLinkLayer/4(snd_param_out) -> Bus Creator/4

== system AtomicLibrary/UserInterface/Link Layer HMI_RESET.master ==
  port_in : Inport  Tag=id=_r-neUPdmEeGH_6eRdlYQdA  Port=1  PortDimensions=-1  DataType=auto  OutDataType=fixdt(1, 16)  OutScaling=2^0  UseBusObject=on  OutDataTypeStr=Inherit: auto
      settings: BusObject=PacketBus
  net_address : Inport  Tag=id=_r-vaIPdmEeGH_6eRdlYQdA  Port=2  PortDimensions=-1  DataType=uint8  OutDataType=fixdt(1, 16)  OutScaling=2^0  OutDataTypeStr=uint8
  receiver_net_address : Inport  Tag=id=_r-woQPdmEeGH_6eRdlYQdA  Port=3  PortDimensions=-1  DataType=uint8  OutDataType=fixdt(1, 16)  OutScaling=2^0  OutDataTypeStr=uint8
  read_event_queue_in : Inport  Tag=id=_r-oFYPdmEeGH_6eRdlYQdA  Port=4  PortDimensions=-1  DataType=auto  OutDataType=fixdt(1, 16)  OutScaling=2^0  OutDataTypeStr=Inherit: auto
  read_event_param_queue_in : Inport  Tag=id=_r-p6kPdmEeGH_6eRdlYQdA  Port=5  PortDimensions=-1  DataType=auto  OutDataType=fixdt(1, 16)  OutScaling=2^0  OutDataTypeStr=Inherit: auto
  read_event_queue_out : Inport  Tag=id=_r-rIsPdmEeGH_6eRdlYQdA  Port=6  PortDimensions=-1  DataType=auto  OutDataType=fixdt(1, 16)  OutScaling=2^0  OutDataTypeStr=Inherit: auto
  read_event_param_queue_out : Inport  Tag=id=_r-sW0PdmEeGH_6eRdlYQdA  Port=7  PortDimensions=-1  DataType=auto  OutDataType=fixdt(1, 16)  OutScaling=2^0  OutDataTypeStr=Inherit: auto
  port_out : Outport  Tag=id=_r-m3QPdmEeGH_6eRdlYQdA  Port=1  PortDimensions=-1  DataType=auto  OutDataType=fixdt(1, 16)  OutScaling=2^0  UseBusObject=on  OutDataTypeStr=Inherit: auto
      settings: BusObject=PacketBus
  write_event_queue_in : Outport  Tag=id=_r-oscPdmEeGH_6eRdlYQdA  Port=2  PortDimensions=-1  DataType=auto  OutDataType=fixdt(1, 16)  OutScaling=2^0  OutDataTypeStr=Inherit: auto
  write_event_param_queue_in : Outport  Tag=id=_r-pTgPdmEeGH_6eRdlYQdA  Port=3  PortDimensions=-1  DataType=auto  OutDataType=fixdt(1, 16)  OutScaling=2^0  OutDataTypeStr=Inherit: auto
  write_event_queue_out : Outport  Tag=id=_r-s94PdmEeGH_6eRdlYQdA  Port=4  PortDimensions=-1  DataType=auto  OutDataType=fixdt(1, 16)  OutScaling=2^0  OutDataTypeStr=Inherit: auto
  write_event_param_queue_out : Outport  Tag=id=_r-uMAPdmEeGH_6eRdlYQdA  Port=5  PortDimensions=-1  DataType=auto  OutDataType=fixdt(1, 16)  OutScaling=2^0  OutDataTypeStr=Inherit: auto
  DataLinkLayer : Subsystem  Tag=id=_r-x2YfdmEeGH_6eRdlYQdA
  Bus Selector : BusSelector  OutputSignals=from,to,msg,param,pkgid,time  Tag=id=_r-xPUPdmEeGH_6eRdlYQdA
  Unit Delay1 : UnitDelay  Tag=id=_r-xPUfdmEeGH_6eRdlYQdA  SampleTime=-1
  Unit Delay2 : UnitDelay  Tag=id=_r-x2YPdmEeGH_6eRdlYQdA  SampleTime=-1
  Unit Delay3 : UnitDelay  Tag=id=_r-ydcPdmEeGH_6eRdlYQdA  SampleTime=-1
  Bus Creator : BusCreator  Inputs=6  UseBusObject=on  Tag=id=_r-ydcfdmEeGH_6eRdlYQdA
      settings: BusObject=PacketBus
  Unit Delay4 : UnitDelay  Tag=id=_r-ydcvdmEeGH_6eRdlYQdA  SampleTime=-1
  Terminator : Terminator
      settings: Tag=id=_r-zEgPdmEeGH_6eRdlYQdA
  Receive Packet : Stateflow chart  Tag=id=_r-zEgfdmEeGH_6eRdlYQdA
  Send Packet : Stateflow chart  Tag=id=_r-zrkPdmEeGH_6eRdlYQdA
  wires:
  DataLinkLayer/3(snd_msg_out) -> Bus Creator/3
  DataLinkLayer/8(recv_msg_out) -> Receive Packet/2(packetMsg)
  Send Packet/3(eventQueue) -> Unit Delay1/1
  DataLinkLayer/7(recv_from_out) -> Receive Packet/1(packetFrom)
  Bus Selector/3 -> DataLinkLayer/3(recv_msg_in)
  read_event_param_queue_in/1 -> Receive Packet/5(eventParamQueueIn)
  Receive Packet/3(bufferOverflow) -> Terminator/1
  receiver_net_address/1 -> DataLinkLayer/8(snd_to_in)
  Receive Packet/2(eventParamQueue) -> Unit Delay4/1
  read_event_queue_out/1 -> Send Packet/2(eventQueueIn)
  DataLinkLayer/9(recv_param_out) -> Receive Packet/3(packetParam)
  Send Packet/2(packetParam) -> DataLinkLayer/10(snd_param_in)
  Bus Selector/2 -> DataLinkLayer/2(recv_to_in)
  port_in/1 -> Bus Selector/1
  read_event_param_queue_out/1 -> Send Packet/3(eventParamQueueIn)
  Send Packet/4(eventParamQueue) -> Unit Delay2/1
  Bus Selector/5 -> DataLinkLayer/5(recv_pkgid_in)
  Unit Delay4/1 -> write_event_param_queue_in/1
  read_event_queue_in/1 -> Receive Packet/4(eventQueueIn)
  Bus Selector/4 -> DataLinkLayer/4(recv_param_in)
  DataLinkLayer/2(snd_to_out) -> Bus Creator/2
  Bus Selector/6 -> DataLinkLayer/6(recv_time_in), Send Packet/1(busSizeSignal)
  Receive Packet/1(eventQueue) -> Unit Delay3/1
  DataLinkLayer/6(snd_time_out) -> Bus Creator/6
  Unit Delay1/1 -> write_event_queue_out/1
  DataLinkLayer/1(snd_from_out) -> Bus Creator/1
  DataLinkLayer/5(snd_pkgid_out) -> Bus Creator/5
  net_address/1 -> DataLinkLayer/7(snd_from_in)
  Send Packet/1(packetMsg) -> DataLinkLayer/9(snd_msg_in)
  Bus Creator/1 -> port_out/1  "Outport13"
  Unit Delay3/1 -> write_event_queue_in/1
  Bus Selector/1 -> DataLinkLayer/1(recv_from_in)
  Unit Delay2/1 -> write_event_param_queue_out/1
  DataLinkLayer/4(snd_param_out) -> Bus Creator/4

== system AtomicLibrary/UserInterface/Link Layer HMI_STRATEGY.master ==
  port_in : Inport  Tag=id=_sIzVEPdmEeGH_6eRdlYQdA  Port=1  PortDimensions=-1  DataType=auto  OutDataType=fixdt(1, 16)  OutScaling=2^0  UseBusObject=on  OutDataTypeStr=Inherit: auto
      settings: BusObject=PacketBus
  net_address : Inport  Tag=id=_sI-7QPdmEeGH_6eRdlYQdA  Port=2  PortDimensions=-1  DataType=uint8  OutDataType=fixdt(1, 16)  OutScaling=2^0  OutDataTypeStr=uint8
  receiver_net_address : Inport  Tag=id=_sJAJYPdmEeGH_6eRdlYQdA  Port=3  PortDimensions=-1  DataType=uint8  OutDataType=fixdt(1, 16)  OutScaling=2^0  OutDataTypeStr=uint8
  read_event_queue_in : Inport  Tag=id=_sI0jMPdmEeGH_6eRdlYQdA  Port=4  PortDimensions=-1  DataType=auto  OutDataType=fixdt(1, 16)  OutScaling=2^0  OutDataTypeStr=Inherit: auto
  read_event_param_queue_in : Inport  Tag=id=_sI3mgPdmEeGH_6eRdlYQdA  Port=5  PortDimensions=-1  DataType=auto  OutDataType=fixdt(1, 16)  OutScaling=2^0  OutDataTypeStr=Inherit: auto
  read_event_queue_out : Inport  Tag=id=_sI40oPdmEeGH_6eRdlYQdA  Port=6  PortDimensions=-1  DataType=auto  OutDataType=fixdt(1, 16)  OutScaling=2^0  OutDataTypeStr=Inherit: auto
  read_event_param_queue_out : Inport  Tag=id=_sI6CwPdmEeGH_6eRdlYQdA  Port=7  PortDimensions=-1  DataType=auto  OutDataType=fixdt(1, 16)  OutScaling=2^0  OutDataTypeStr=Inherit: auto
  port_out : Outport  Tag=id=_sIyuAfdmEeGH_6eRdlYQdA  Port=1  PortDimensions=-1  DataType=auto  OutDataType=fixdt(1, 16)  OutScaling=2^0  UseBusObject=on  OutDataTypeStr=Inherit: auto
      settings: BusObject=PacketBus
  write_event_queue_in : Outport  Tag=id=_sI1KQPdmEeGH_6eRdlYQdA  Port=2  PortDimensions=-1  DataType=auto  OutDataType=fixdt(1, 16)  OutScaling=2^0  OutDataTypeStr=Inherit: auto
  write_event_param_queue_in : Outport  Tag=id=_sI2YYPdmEeGH_6eRdlYQdA  Port=3  PortDimensions=-1  DataType=auto  OutDataType=fixdt(1, 16)  OutScaling=2^0  OutDataTypeStr=Inherit: auto
  write_event_queue_out : Outport  Tag=id=_sI7Q4PdmEeGH_6eRdlYQdA  Port=4  PortDimensions=-1  DataType=auto  OutDataType=fixdt(1, 16)  OutScaling=2^0  OutDataTypeStr=Inherit: auto
  write_event_param_queue_out : Outport  Tag=id=_sI8fAPdmEeGH_6eRdlYQdA  Port=5  PortDimensions=-1  DataType=auto  OutDataType=fixdt(1, 16)  OutScaling=2^0  OutDataTypeStr=Inherit: auto
  DataLinkLayer : Subsystem  Tag=id=_sJClovdmEeGH_6eRdlYQdA
  Bus Selector : BusSelector  OutputSignals=from,to,msg,param,pkgid,time  Tag=id=_sJB-kPdmEeGH_6eRdlYQdA
  Unit Delay1 : UnitDelay  Tag=id=_sJCloPdmEeGH_6eRdlYQdA  SampleTime=-1
  Unit Delay2 : UnitDelay  Tag=id=_sJClofdmEeGH_6eRdlYQdA  SampleTime=-1
  Unit Delay3 : UnitDelay  Tag=id=_sJDMsPdmEeGH_6eRdlYQdA  SampleTime=-1
  Bus Creator : BusCreator  Inputs=6  UseBusObject=on  Tag=id=_sJDMsfdmEeGH_6eRdlYQdA
      settings: BusObject=PacketBus
  Unit Delay4 : UnitDelay  Tag=id=_sJDzwPdmEeGH_6eRdlYQdA  SampleTime=-1
  Terminator : Terminator
      settings: Tag=id=_sJDzwfdmEeGH_6eRdlYQdA
  Receive Packet : Stateflow chart  Tag=id=_sJDzwvdmEeGH_6eRdlYQdA
  Send Packet : Stateflow chart  Tag=id=_sJEa0PdmEeGH_6eRdlYQdA
  wires:
  DataLinkLayer/3(snd_msg_out) -> Bus Creator/3
  DataLinkLayer/8(recv_msg_out) -> Receive Packet/2(packetMsg)
  Send Packet/3(eventQueue) -> Unit Delay1/1
  DataLinkLayer/7(recv_from_out) -> Receive Packet/1(packetFrom)
  Bus Selector/3 -> DataLinkLayer/3(recv_msg_in)
  read_event_param_queue_in/1 -> Receive Packet/5(eventParamQueueIn)
  Receive Packet/3(bufferOverflow) -> Terminator/1
  receiver_net_address/1 -> DataLinkLayer/8(snd_to_in)
  Receive Packet/2(eventParamQueue) -> Unit Delay4/1
  read_event_queue_out/1 -> Send Packet/2(eventQueueIn)
  DataLinkLayer/9(recv_param_out) -> Receive Packet/3(packetParam)
  Send Packet/2(packetParam) -> DataLinkLayer/10(snd_param_in)
  Bus Selector/2 -> DataLinkLayer/2(recv_to_in)
  port_in/1 -> Bus Selector/1
  read_event_param_queue_out/1 -> Send Packet/3(eventParamQueueIn)
  Send Packet/4(eventParamQueue) -> Unit Delay2/1
  Bus Selector/5 -> DataLinkLayer/5(recv_pkgid_in)
  Unit Delay4/1 -> write_event_param_queue_in/1
  read_event_queue_in/1 -> Receive Packet/4(eventQueueIn)
  Bus Selector/4 -> DataLinkLayer/4(recv_param_in)
  DataLinkLayer/2(snd_to_out) -> Bus Creator/2
  Bus Selector/6 -> DataLinkLayer/6(recv_time_in), Send Packet/1(busSizeSignal)
  Receive Packet/1(eventQueue) -> Unit Delay3/1
  DataLinkLayer/6(snd_time_out) -> Bus Creator/6
  Unit Delay1/1 -> write_event_queue_out/1
  DataLinkLayer/1(snd_from_out) -> Bus Creator/1
  DataLinkLayer/5(snd_pkgid_out) -> Bus Creator/5
  net_address/1 -> DataLinkLayer/7(snd_from_in)
  Send Packet/1(packetMsg) -> DataLinkLayer/9(snd_msg_in)
  Bus Creator/1 -> port_out/1  "Outport15"
  Unit Delay3/1 -> write_event_queue_in/1
  Bus Selector/1 -> DataLinkLayer/1(recv_from_in)
  Unit Delay2/1 -> write_event_param_queue_out/1
  DataLinkLayer/4(snd_param_out) -> Bus Creator/4
